simulink model "dc_motor_PID"  (R2024b)
settings: Solver=VariableStepAuto  StartTime=0.0  StopTime=10.0  RelTol=1e-3
PreLoadFcn:
  | load properties.mat
values from neighbouring files (symbols this model uses):
  b = 0.1    [properties.mat]
  J = 0.01    [properties.mat]
  K = 0.1    [properties.mat]
  L = 0.5    [properties.mat]
  R = 1    [properties.mat]
libraries: slpidlib x1
settings Model: Creator=garellan  LastModifiedBy=garellan

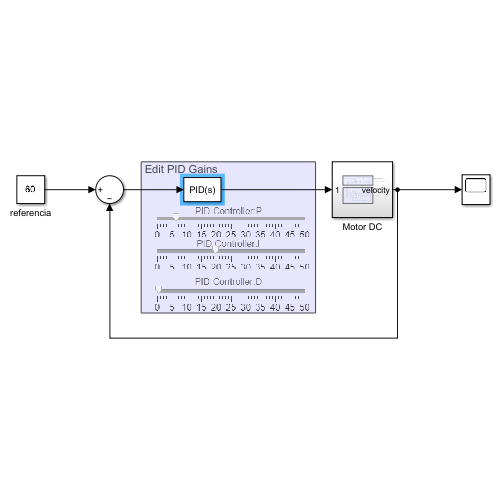
[thumbnail: Simulink's stored preview of the top-level diagram]
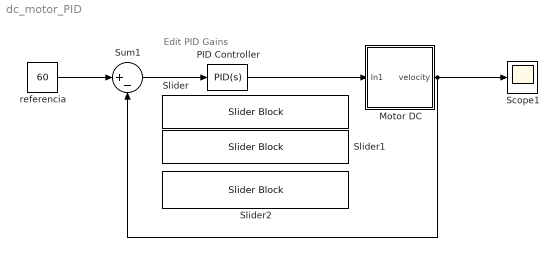
== system dc_motor_PID ==
  note: Edit PID Gains
  Motor DC : Subsystem
  PID Controller : slpidlib/PID Controller  Controller=PID  Form=Parallel  TimeDomain=Continuous-time  UseExternalTs=off  SampleTime=-1  IntegratorMethod=Forward Euler  FilterMethod=Forward Euler  ControllerParametersSource=internal  P=6.39716081653734  I=19.9057154618901  UseKiTs=off  D=0.444004423077837  UseExternalDerivativeSource=off  N=105.867340373296  UseFilter=on  TunerSelectOption=Transfer Function Based (PID Tuner App)  InitialConditionSource=internal  InitialConditionForIntegrator=0  InitialConditionForFilter=0  DifferentiatorICPrevScaledInput=0  ExternalReset=none  TrackingMode=off  Kt=1  LimitOutput=off  SatLimitsSource=internal  UpperSaturationLimit=inf  LowerSaturationLimit=-inf  LinearizeAsGain=on  AntiWindupMode=none  Kb=1  LimitIntegrator=off  UpperIntegratorSaturationLimit=inf  LowerIntegratorSaturationLimit=-inf  POutMin=[]  POutMax=[]  IOutMin=[]  IOutMax=[]  DOutMin=[]  DOutMax=[]  NOutMin=[]  NOutMax=[]  SumOutMin=[]  SumOutMax=[]  SaturationOutMin=[]  SaturationOutMax=[]  PParamMin=[]  PParamMax=[]  IParamMin=[]  IParamMax=[]  DParamMin=[]  DParamMax=[]  NParamMin=[]  NParamMax=[]  KbParamMin=[]  KbParamMax=[]  KtParamMin=[]  KtParamMax=[]  KbOutMin=[]  KbOutMax=[]  KtOutMin=[]  KtOutMax=[]  IntegratorOutMin=[]  IntegratorOutMax=[]  FilterOutMin=[]  FilterOutMax=[]  SumI1OutMin=[]  SumI1OutMax=[]  SumI2OutMin=[]  SumI2OutMax=[]  SumI3OutMin=[]  SumI3OutMax=[]  SumI4OutMin=[]  SumI4OutMax=[]  SumDOutMin=[]  SumDOutMax=[]  DifferentiatorOutMin=[]  DifferentiatorOutMax=[]  FilterDiffOutCoefMin=[]  FilterDiffOutCoefMax=[]  ReciprocalOutMin=[]  ReciprocalOutMax=[]  SumDenOutMin=[]  SumDenOutMax=[]  SumNumOutMin=[]  SumNumOutMax=[]  DivideOutMin=[]  DivideOutMax=[]  UdiffTsProdOutMin=[]  UdiffTsProdOutMax=[]  NTsProdOutMin=[]  NTsProdOutMax=[]  UintegralTsProdOutMin=[]  UintegralTsProdOutMax=[]  UngainTsProdOutMin=[]  UngainTsProdOutMax=[]  ClampingZeroOutDataTypeStr=Inherit: Inherit via back propagation  ClampingZeroOutMin=[]  ClampingZeroOutMax=[]  FilterDenConstantOutDataTypeStr=Inherit: Inherit via back propagation  FilterDenConstantOutMin=[]  FilterDenConstantOutMax=[]  PCopyOutDataTypeStr=Inherit: Inherit via back propagation  PCopyOutMin=[]  PCopyOutMax=[]  NCopyOutDataTypeStr=Inherit: Inherit via back propagation  NCopyOutMin=[]  NCopyOutMax=[]  IntegratorContinuousStateAttributes=''  IntegratorStateMustResolveToSignalObject=off  IntegratorRTWStateStorageClass=Auto  FilterContinuousStateAttributes=''  FilterStateMustResolveToSignalObject=off  FilterRTWStateStorageClass=Auto  ParallelPVariant=InternalParameters  IdealPVariant=Disabled  IVariant=InternalParameters  DVariant=InternalParameters  IntegratorVariant=Continuous  SatVariant=Disabled  AWVariant=Passthrough  PCopyVariant=Disabled  TRVariant=Disabled  FdbkBlocksVariant=Forward  IdealPFdbkVariant=Disabled  SatFdbkVariant=Disabled  DerivativeFilterVariant=ContFilter  NVariant=InternalParameters  NCopyVariant=Disabled  FilterICVariant=InternalICsFilter  IntegratorICVariant=InternalICs  ExternalResetVariant=Disabled  TRSumVariant=Passthrough  SumFdbkVariant=Disabled  SumVariant=Sum_PID  TsampFilterVariant=InternalTs  TsampNgainVariant=Passthrough  TsampIntegralVariant=Disabled_SignalSpec  ExternalSaturationOutDataTypeStr=Inherit: Same as second input  DerivativeSourceVariant=ErrorSignal  PreIntVariant=InternalPreInt
  Scope1 : Scope
  Slider : SliderBlock  ScaleMax=50
  Slider1 : SliderBlock  ScaleMax=50
  Slider2 : SliderBlock  ScaleMax=50
  Sum1 : Sum  Inputs=|+-
  referencia : Constant  Value=60
  wires:
  PID Controller/1 -> Motor DC/1(In1)
  referencia/1 -> Sum1/1
  Sum1/1 -> PID Controller/1
  Motor DC/1(velocity) -> Scope1/1, Sum1/2

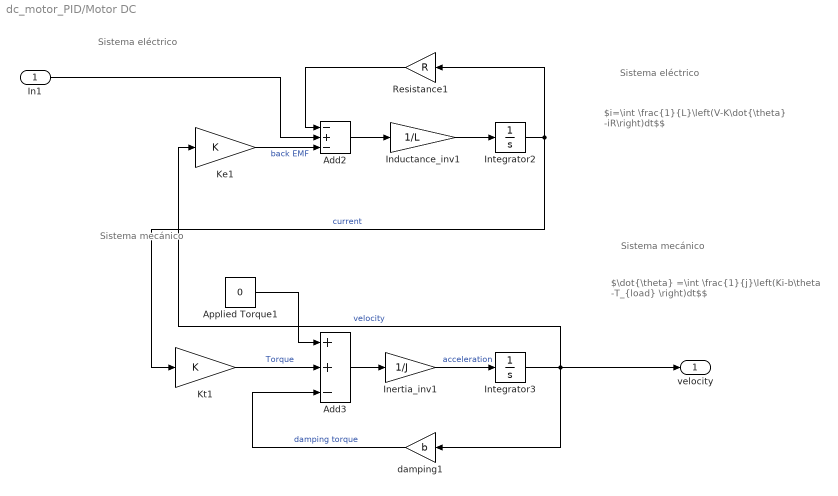
== system dc_motor_PID/Motor DC ==
  note: Sistema eléctrico
  note: Sistema mecánico
  note: $\dot{\theta} =\int \frac{1}{j}\left(Ki-b\theta -T_{load} \right)dt$$
  note: Sistema mecánico
  note: $i=\int \frac{1}{L}\left(V-K\dot{\theta} -iR\right)dt$$
  note: Sistema eléctrico
  In1 : Inport
  Add2 : Sum  Inputs=-+-
  Add3 : Sum  Inputs=++-
  Applied Torque1 : Constant  Value=0
  Inductance_inv1 : Gain  Gain=1/L
  Inertia_inv1 : Gain  Gain=1/J
  Integrator2 : Integrator
  Integrator3 : Integrator
  Ke1 : Gain  Gain=K
  Kt1 : Gain  Gain=K
  Resistance1 : Gain  Gain=R
  damping1 : Gain  Gain=b
  velocity : Outport
  wires:
  Applied Torque1/1 -> Add3/1
  Integrator2/1 -> Kt1/1, Resistance1/1  "current"
  damping1/1 -> Add3/3  "damping torque"
  Integrator3/1 -> velocity/1, Ke1/1, damping1/1  "velocity"
  Resistance1/1 -> Add2/1
  Inductance_inv1/1 -> Integrator2/1
  Add2/1 -> Inductance_inv1/1
  Inertia_inv1/1 -> Integrator3/1  "acceleration"
  Ke1/1 -> Add2/3  "back EMF"
  Add3/1 -> Inertia_inv1/1
  Kt1/1 -> Add3/2  "Torque"
  In1/1 -> Add2/2
